simulink model "Five_Level_Cascaded_H_Bridge_CHB_Multilevel_Inverter"  (R2023b)
settings: Solver=VariableStepAuto  StartTime=0.0  StopTime=0.1  RelTol=1e-3
libraries: spsIGBTLib x8, simulink x4, spsDCVoltageSourceLib x2, spsVoltageMeasurementLib x1, sps_lib x1
settings Model: Creator=HP  LastModifiedBy=HP

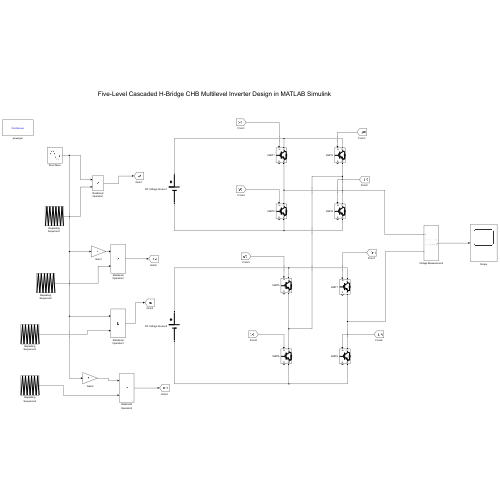
[thumbnail: Simulink's stored preview of the top-level diagram]
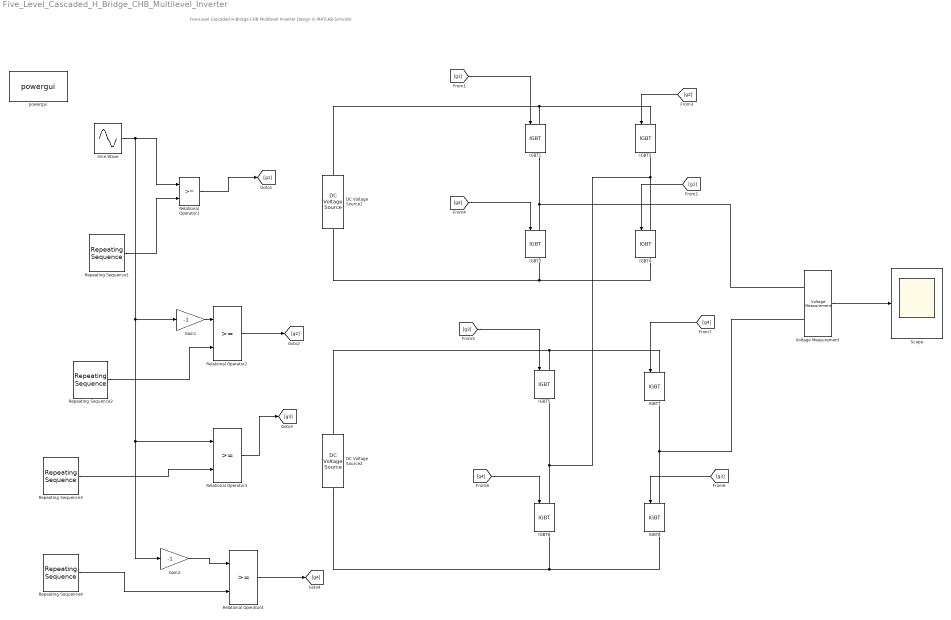
== system Five_Level_Cascaded_H_Bridge_CHB_Multilevel_Inverter ==
  note: Five-Level Cascaded H-Bridge CHB Multilevel Inverter Design in MATLAB Simulink
  DC Voltage Source1 : spsDCVoltageSourceLib/DC Voltage Source  Amplitude=100  Measurements=None
  DC Voltage Source2 : spsDCVoltageSourceLib/DC Voltage Source  Amplitude=100  Measurements=None
  Gain1 : Gain  Gain=-1
  Gain2 : Gain  Gain=-1
  IGBT{1..8} (8 alike) : spsIGBTLib/IGBT  Ron=0.001  Lon=0  Vf=1  Tf=1e-6  Tt=2e-6  IC=0  Rs=1e5  Cs=inf  Measurements=on
  Relational Operator{1..4} (4 alike) : RelationalOperator  OutDataTypeStr=boolean  RndMeth=Simplest  InputSameDT=off
  Repeating Sequence1 : simulink/Sources/Repeating Sequence  rep_seq_t=[0 1e-3 0.002 0.003 0.004]  rep_seq_y=[0 1 0 1 0]
  Repeating Sequence2 : simulink/Sources/Repeating Sequence  rep_seq_t=[0 1e-3 0.002 0.003 0.004]  rep_seq_y=[0 1 0 1 0]
  Repeating Sequence3 : simulink/Sources/Repeating Sequence  rep_seq_t=[0 1e-3 0.002 0.003 0.004]  rep_seq_y=[1 2 1 2 1]
  Repeating Sequence4 : simulink/Sources/Repeating Sequence  rep_seq_t=[0 1e-3 0.002 0.003 0.004]  rep_seq_y=[1 2 1 2 1]
  Scope : Scope
  Sine Wave : Sin  Amplitude=2  Frequency=2*pi*50  SampleTime=0
  Voltage Measurement : spsVoltageMeasurementLib/Voltage Measurement  PhasorSimulation=off  OutputType=Complex  PSBequivalent=0
  powergui : sps_lib/powergui  Priority=1  SimulationMode=Continuous  SampleTime=50e-6  frequency=60  Iterations=50  frequencyindice=0  Pbase=100e6  ErrMax=1e-4  UnitsV=kV  UnitsW=MW  buscounter=0  FunctionMessages=off  echomessages=off  EnableUseOfTLC=off  CurrentSourceSwitches=off  DisableSnubberDevices=off  DisableRonSwitches=off  DisableVfSwitches=off  DisplayEquations=off  AutomaticDiscreteSolvers=off  SolverType=Tustin/Backward Euler (TBE)  Interpol=off  ExternalGateDelay=off  methode=off  Ts=100  x0status=blocks  SPID=on  SwTol=0  HookPort=off  NonlinearTolerance=1e-4  nMaxIteration=100  ContinueOnMaxIteration=off  RestoreLinks=warning  ResistiveCurrentMeasurement=off  Frange=[0:2:500]  Ylog=off  Xlog=on  ShowGrid=off  save=off  variable=ZData  structure=0  ZoomFFT=off  StartTime=0.0  cycles=1  DisplayStyle=1  fundamental=60  FreqAxis=off  MaxFrequency=1000  frequencyindicesteady=1  RmsSteady=1  display=off
  wires:
  [g1] -> IGBT1/1
  [g1] -> IGBT4/1
  [g2] -> IGBT3/1
  [g2] -> IGBT2/1
  [g3] -> IGBT5/1
  [g3] -> IGBT8/1
  [g4] -> IGBT7/1
  [g4] -> IGBT6/1
  Relational Operator1/1 -> [g1]
  Sine Wave/1 -> Gain1/1, Gain2/1, Relational Operator3/1, Relational Operator1/1
  Repeating Sequence1/1 -> Relational Operator1/2
  Gain1/1 -> Relational Operator2/1
  Repeating Sequence2/1 -> Relational Operator2/2
  Relational Operator2/1 -> [g2]
  Relational Operator3/1 -> [g3]
  Repeating Sequence3/1 -> Relational Operator3/2
  Gain2/1 -> Relational Operator4/1
  Relational Operator4/1 -> [g4]
  Repeating Sequence4/1 -> Relational Operator4/2
  Voltage Measurement/1 -> Scope/1
  connections:
  IGBT1/RConn1 -- Voltage Measurement/LConn1 -- IGBT2/LConn1
  IGBT1/LConn1 -- DC Voltage Source1/RConn1 -- IGBT3/LConn1
  IGBT4/RConn1 -- DC Voltage Source1/LConn1 -- IGBT2/RConn1
  IGBT6/LConn1 -- IGBT5/RConn1 -- IGBT4/LConn1 -- IGBT3/RConn1
  IGBT8/LConn1 -- Voltage Measurement/LConn2 -- IGBT7/RConn1
  IGBT5/LConn1 -- DC Voltage Source2/RConn1 -- IGBT7/LConn1
  IGBT8/RConn1 -- DC Voltage Source2/LConn1 -- IGBT6/RConn1
